simulink model "control_system"  (R2016b)
settings: Solver=FixedStepDiscrete  StartTime=0.0  StopTime=inf  FixedStep=0.004  MaxStep=0.004  RelTol=1e-3
undefined symbols (not defined in the file or in its folder): DiscIntNeverNeededParam
libraries: simulink x11
settings Model: Creator=ADAM  LastModifiedBy=consti
settings SolverCC: ExtrapolationOrder=1
settings DataIOCC: MaxDataPoints=1  SaveFormat=Structure  SignalLoggingSaveFormat=ModelDataLogs  SaveOutput=off  DSMLogging=off  SaveTime=off  OutputSaveName=model_out  SignalLoggingName=model_out
settings OptimizationCC: DefaultParameterBehavior=Inlined  UseFloatMulNetSlope=on  InlineInvariantSignals=on  PassReuseOutputArgsAs=Individual arguments  ExpressionDepthLimit=2147483647  ZeroExternalMemoryAtStartup=off  ZeroInternalMemoryAtStartup=off  NoFixptDivByZeroProtection=on  EfficientFloat2IntCast=on  LifeSpan=1
settings DebuggingCC: UnderspecifiedInitializationDetection=Classic  MergeDetectMultiDrivingBlocksExec=none  SolverPrmCheckMsg=warning  InheritedTsInSrcMsg=none  MultiTaskDSMMsg=warning  MultiTaskCondExecSysMsg=none  ParameterTunabilityLossMsg=error  UnconnectedInputMsg=none  UnconnectedOutputMsg=none  UnconnectedLineMsg=none  StateNameClashWarn=warning  SFUnexpectedBacktrackingDiag=warning  SFNoUnconditionalDefaultTransitionDiag=warning  SFExecutionAtInitializationDiag=none
settings HardwareCC: ProdBitPerLong=64  ProdHWDeviceType=Intel->x86-64 (Linux 64)
settings ModelReferenceCC: PropagateSignalLabelsOutOfModel=off
settings RTWCC: SystemTargetFile=ert.tlc  TemplateMakefile=ert_default_tmf  Description=Embedded Coder  GenerateReport=on  IncludeHyperlinkInReport=on  LaunchReport=on  GenerateTraceInfo=on  GenerateTraceReport=on  GenerateTraceReportSl=on  GenerateTraceReportSf=on  GenerateTraceReportEml=on  GenerateCodeMetricsReport=on
settings CodeAppCC: ForceParamTrailComments=on  IgnoreCustomStorageClasses=off  MaxIdLength=95  OperatorAnnotations=on  SimulinkDataObjDesc=on  SFDataObjDesc=on  MATLABFcnDesc=on  CustomSymbolStrGlobalVar=rt$N$M  CustomSymbolStrType=$N$M  CustomSymbolStrFcn=$N$M$F  CustomSymbolStrMacro=$N$M  InsertBlockDesc=on  MATLABSourceComments=on
settings ERTTargetCC: GenerateSampleERTMain=on  CombineSignalStateStructs=on  SupportAbsoluteTime=off  SupportComplex=off  SupportNonInlinedSFcns=on  InlinedParameterPlacement=NonHierarchical  ERTCustomFileTemplate=example_file_process.tlc  ERTFilePackagingFormat=CompactWithDataFile
settings ConfigComp: CovMetricSettings=dw  CovHtmlReporting=on  CovSaveCumulativeToWorkspaceVar=on  CovSaveSingleToWorkspaceVar=on  CovExternalEMLEnable=off  CovSFcnEnable=off

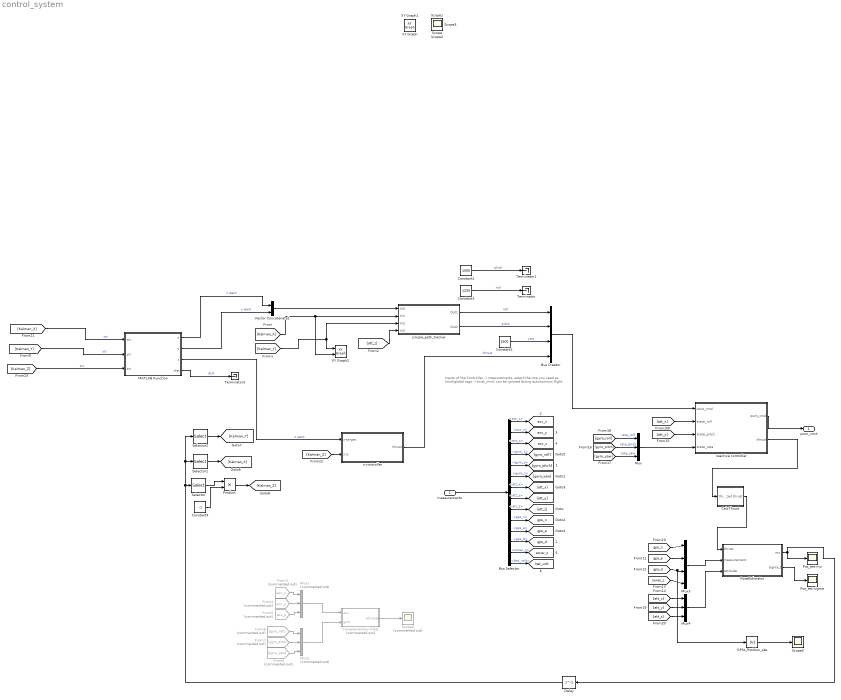
== system control_system ==
  note: Inputs of the Controller
      | -) measurements: select the one you need as local/global tags
      | -) twist_cmd: can be ignored during autonomous flight
  measurements : Inport  OutDataTypeStr=Bus: Sensor_Bus  SampleTime=[0.0040000000000000001,0]
  Bus Creator : BusCreator  Inputs=4
  Bus Selector : BusSelector  OutputSignals=acc_x,acc_y,acc_z,gyro_x,gyro_y,gyro_z,att_x,att_y,att_z,gps_n,gps_e,gps_d,sonar_z,bat_volt
  "CalcThrust " : MATLAB Function  TreatAsAtomicUnit=on
  Complementary Filter : Subsystem  Commented=on
  Constant1 : Constant  Value=1500
  Constant2 : Constant  Value=1500
  Constant3 : Constant  Value=1250
  Constant4 : Constant  Value=-1
  Delay : Delay  DelayLength=1  InitialCondition=0
  From3 : From  Commented=on  GotoTag=acc_x  TagVisibility=global
  From4 : From  Commented=on  GotoTag=acc_y  TagVisibility=global
  From5 : From  Commented=on  GotoTag=acc_z  TagVisibility=global
  From6 : From  Commented=on  GotoTag=gyro_roll
  From7 : From  Commented=on  GotoTag=gyro_pitch
  From8 : From  Commented=on  GotoTag=gyro_yaw
  GPSz_Position_abs : Abs
  MATLAB Function : MATLAB Function  TreatAsAtomicUnit=on
  Mux : Mux  Inputs=3
  Mux1 : Mux  Commented=on  Inputs=3
  Mux2 : Mux  Commented=on  Inputs=3
  Mux3 : Mux
  Mux4 : Mux  Inputs=3
  Pos_est-mu : Scope
  Pos_est-sigma : Scope
  "PoseEstimator " : MATLAB Function  TreatAsAtomicUnit=on
  Product : Product
  Scope4 : Scope  Commented=on
  Scope{,1..3,5} (5 alike) : Scope
  Selector : Selector  InputPortWidth=6  IndexOptions=Index vector (dialog)  Indices=[3]  OutputSizes=1
  Selector1 : Selector  InputPortWidth=6  IndexOptions=Index vector (dialog)  Indices=[2]  OutputSizes=1
  Selector2 : Selector  InputPortWidth=6  IndexOptions=Index vector (dialog)  Indices=[1]  OutputSizes=1
  Terminator : Terminator
  Terminator1 : Terminator
  Terminator3 : Terminator
  Vector Concatenate1 : Concatenate
  XY Graph2 : simulink/Sinks/XY Graph  xmin=0  xmax=20  ymin=0  ymax=20  st=-1
  reactive controller : Subsystem  TreatAsAtomicUnit=on
  "simple_path_tracker " : Subsystem
  z-controller : Subsystem
  pwm_cmd : Outport  OutDataTypeStr=Bus: Motor_Bus  SampleTime=[0.0040000000000000001,0]
  XY Graph : simulink/Sinks/XY Graph  IOType=viewer  xmin=-1  xmax=1  ymin=-1  ymax=1  st=-1
  XY Graph1 : simulink/Sinks/XY Graph  IOType=viewer  xmin=-1  xmax=1  ymin=-1  ymax=1  st=-1
  tag scope: acc_x=global, acc_y=global, acc_z=global, bat_volt=global, gps_d=global, gps_e=global, gps_n=global, sonar_z=global
  wires:
  reactive controller/1(pwm_cmd) -> pwm_cmd/1
  measurements/1 -> Bus Selector/1
  Mux/1 -> reactive controller/4(state_rate)
  [gyro_yaw] -> Mux/3  "rate_yaw"
  [gyro_pitch] -> Mux/2  "rate_pitch"
  [gyro_roll] -> Mux/1  "rate_roll"
  [att_y] -> reactive controller/3(state_pitch)
  [att_x] -> reactive controller/2(state_roll)
  Bus Selector/1 -> [acc_x]  "<acc_x>"
  Bus Selector/2 -> [acc_y]  "<acc_y>"
  Bus Selector/3 -> [acc_z]  "<acc_z>"
  Bus Selector/7 -> [att_x]  "<att_x>"
  Bus Selector/8 -> [att_y]  "<att_y>"
  Bus Selector/9 -> [att_z]  "<att_z>"
  Bus Selector/10 -> [gps_n]  "<gps_n>"
  Bus Selector/11 -> [gps_e]  "<gps_e>"
  Bus Selector/12 -> [gps_d]  "<gps_d>"
  Bus Selector/13 -> [sonar_z]  "<sonar_z>"
  Bus Selector/14 -> [bat_volt]  "<bat_volt>"
  Bus Selector/4 -> [gyro_roll]  "<gyro_x>"
  Bus Selector/5 -> [gyro_pitch]  "<gyro_y>"
  Bus Selector/6 -> [gyro_yaw]  "<gyro_z>"
  Bus Creator/1 -> reactive controller/1(twist_cmd)
  Constant1/1 -> Bus Creator/3  "yaw"
  z-controller/1(thrust) -> Bus Creator/4  "thrust"
  Vector Concatenate1/1 -> "simple_path_tracker "/1(In4)
  MATLAB Function/1(x) -> Vector Concatenate1/1  "x want"
  [Kalman_X] -> "simple_path_tracker "/2(In1), XY Graph2/2
  [Kalman_Y] -> "simple_path_tracker "/3(In2), XY Graph2/1
  MATLAB Function/2(y) -> Vector Concatenate1/2  "y want"
  [att_z] -> "simple_path_tracker "/4(In3)
  From3/1 -> Mux1/1
  From4/1 -> Mux1/2
  From5/1 -> Mux1/3
  Mux1/1 -> Complementary Filter/1(acc)
  From6/1 -> Mux2/1
  From7/1 -> Mux2/2
  From8/1 -> Mux2/3
  Mux2/1 -> Complementary Filter/2(gyro)
  Complementary Filter/1(attitude) -> Scope4/1
  MATLAB Function/3(z) -> z-controller/1(z-target)  "z want"
  [gps_n] -> Mux3/1
  [gps_e] -> Mux3/2
  [sonar_z] -> Mux3/4
  Mux3/1 -> "PoseEstimator "/2(measurement)
  [att_y] -> Mux4/2
  [att_x] -> Mux4/1
  [att_z] -> Mux4/3
  Mux4/1 -> "PoseEstimator "/3(attitude)
  "PoseEstimator "/2(sigma_t) -> Pos_est-sigma/1
  "CalcThrust "/1(thrust) -> "PoseEstimator "/1(thrust)
  reactive controller/2(thrust) -> "CalcThrust "/1(thrust_normalized)
  [gps_d] -> GPSz_Position_abs/1, Mux3/3
  GPSz_Position_abs/1 -> Scope5/1
  "PoseEstimator "/1(mu) -> Pos_est-mu/1, Delay/1
  Delay/1 -> Selector2/1, Selector1/1, Selector/1
  Selector/1 -> Product/1
  Constant4/1 -> Product/2
  Constant2/1 -> Terminator1/1  "pitch"
  Constant3/1 -> Terminator/1  "roll"
  [Kalman_Y] -> MATLAB Function/2(yis)  "yis"
  [Kalman_X] -> MATLAB Function/1(xis)  "xis"
  [Kalman_Z] -> MATLAB Function/3(zis)  "zis"
  "simple_path_tracker "/1(Out1) -> Bus Creator/1  "roll"
  "simple_path_tracker "/2(Out2) -> Bus Creator/2  "pitch"
  MATLAB Function/4(dist) -> Terminator3/1  "dist"
  Selector1/1 -> [Kalman_X]
  Selector2/1 -> [Kalman_Y]
  Product/1 -> [Kalman_Z]
  [Kalman_Z] -> z-controller/2(z-is)

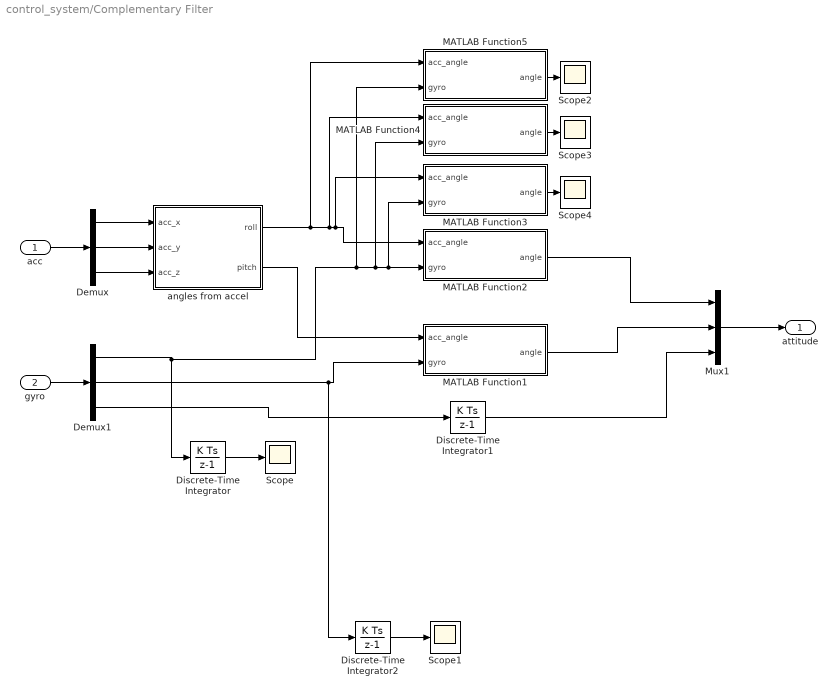
== system control_system/Complementary Filter ==
  acc : Inport  PortDimensions=3
  gyro : Inport  Port=2
  Demux : Demux  Outputs=3
  Demux1 : Demux  Outputs=3
  Discrete-Time Integrator : DiscreteIntegrator  InitialConditionSetting=State (most efficient)  SampleTime=-1  ICPrevOutput=DiscIntNeverNeededParam  ICPrevScaledInput=DiscIntNeverNeededParam
  Discrete-Time Integrator1 : DiscreteIntegrator  InitialConditionSetting=State (most efficient)  SampleTime=-1  ICPrevOutput=DiscIntNeverNeededParam  ICPrevScaledInput=DiscIntNeverNeededParam
  Discrete-Time Integrator2 : DiscreteIntegrator  InitialConditionSetting=State (most efficient)  SampleTime=-1  ICPrevOutput=DiscIntNeverNeededParam  ICPrevScaledInput=DiscIntNeverNeededParam
  MATLAB Function1 : MATLAB Function  TreatAsAtomicUnit=on
  MATLAB Function2 : MATLAB Function  TreatAsAtomicUnit=on
  MATLAB Function3 : MATLAB Function  TreatAsAtomicUnit=on
  MATLAB Function4 : MATLAB Function  TreatAsAtomicUnit=on
  MATLAB Function5 : MATLAB Function  TreatAsAtomicUnit=on
  Mux1 : Mux  Inputs=3
  Scope{,1..4} (5 alike) : Scope
  angles from accel : MATLAB Function  TreatAsAtomicUnit=on
  attitude : Outport
  wires:
  Mux1/1 -> attitude/1
  acc/1 -> Demux/1
  gyro/1 -> Demux1/1
  Demux/1 -> angles from accel/1(acc_x)
  Demux/3 -> angles from accel/3(acc_z)
  Demux/2 -> angles from accel/2(acc_y)
  angles from accel/2(pitch) -> MATLAB Function1/1(acc_angle)
  MATLAB Function1/1(angle) -> Mux1/2
  Discrete-Time Integrator/1 -> Scope/1
  angles from accel/1(roll) -> MATLAB Function5/1(acc_angle), MATLAB Function4/1(acc_angle), MATLAB Function3/1(acc_angle), MATLAB Function2/1(acc_angle)
  MATLAB Function2/1(angle) -> Mux1/1
  Demux1/3 -> Discrete-Time Integrator1/1
  Discrete-Time Integrator1/1 -> Mux1/3
  Demux1/2 -> Discrete-Time Integrator2/1, MATLAB Function1/2(gyro)
  Discrete-Time Integrator2/1 -> Scope1/1
  Demux1/1 -> MATLAB Function5/2(gyro), MATLAB Function4/2(gyro), MATLAB Function2/2(gyro), MATLAB Function3/2(gyro), Discrete-Time Integrator/1
  MATLAB Function5/1(angle) -> Scope2/1
  MATLAB Function4/1(angle) -> Scope3/1
  MATLAB Function3/1(angle) -> Scope4/1

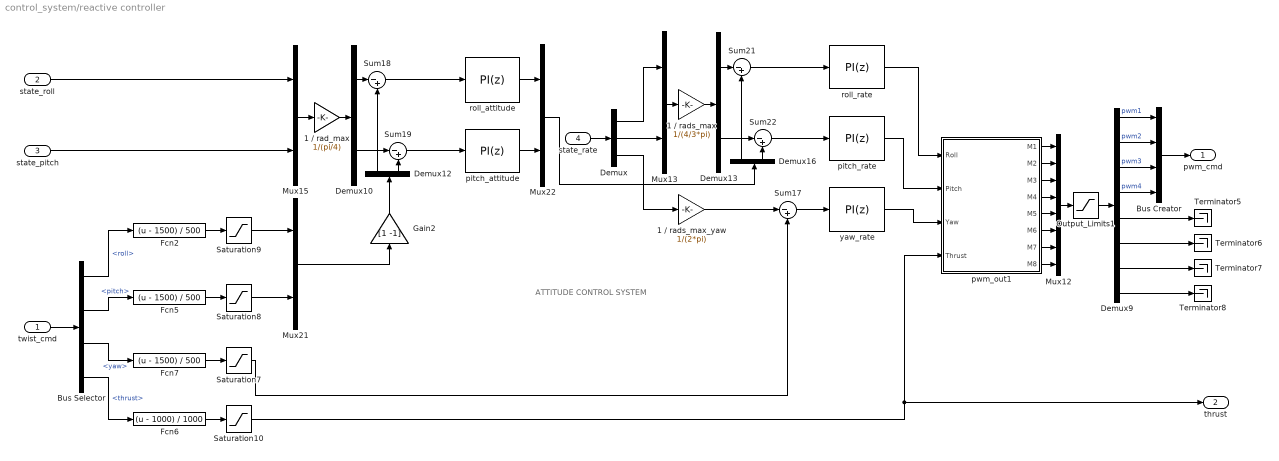
== system control_system/reactive controller ==
  note: ATTITUDE CONTROL SYSTEM
  twist_cmd : Inport  OutDataTypeStr=Bus: Twist_Bus
  state_roll : Inport  Port=2
  state_pitch : Inport  Port=3
  state_rate : Inport  Port=4
  1 / rad_max : Gain  Gain=1/(pi/4)
  1 / rads_max : Gain  Gain=1/(4/3*pi)
  1 / rads_max_yaw : Gain  Gain=1/(2*pi)
  Bus Creator : BusCreator  Inputs=4
  Bus Selector : BusSelector  OutputSignals=roll,pitch,yaw,thrust
  Demux : Demux  Outputs=3
  Demux{10,12..13,16} (4 alike) : Demux  Outputs=2
  Demux9 : Demux  Outputs=8
  Fcn2 : Fcn  Expr=(u - 1500) / 500
  Fcn5 : Fcn  Expr=(u - 1500) / 500
  Fcn6 : Fcn  Expr=(u - 1000) / 1000
  Fcn7 : Fcn  Expr=(u - 1500) / 500
  Gain2 : Gain  Gain=[1 -1]
  Mux12 : Mux  Inputs=8
  Mux{13,15,21..22} (4 alike) : Mux  Inputs=2
  Output_Limits1 : Saturate  UpperLimit=2000  LowerLimit=1000
  Saturation10 : Saturate  UpperLimit=1  LowerLimit=0
  Saturation7 : Saturate  UpperLimit=1  LowerLimit=-1
  Saturation8 : Saturate  UpperLimit=1  LowerLimit=-1
  Saturation9 : Saturate  UpperLimit=1  LowerLimit=-1
  Sum{17..19,21..22} (5 alike) : Sum  Inputs=|-+
  Terminator{5..8} (4 alike) : Terminator
  pitch_attitude : simulink/Continuous/PID Controller  Controller=PI  TimeDomain=Discrete-time  SampleTime=-1  IntegratorMethod=Forward Euler  FilterMethod=Forward Euler  Form=Parallel  UseFilter=on  ControllerParametersSource=internal  P=0.5  I=0.05  D=0.01  N=100  InitialConditionSource=internal  InitialConditionForIntegrator=0  InitialConditionForFilter=0  ExternalReset=none  LimitOutput=on  UpperSaturationLimit=1  LowerSaturationLimit=-1  LinearizeAsGain=on  AntiWindupMode=none  Kb=1  TrackingMode=off  Kt=1  PParamMin=[]  PParamMax=[]  IParamMin=[]  IParamMax=[]  DParamMin=[]  DParamMax=[]  NParamMin=[]  NParamMax=[]  KbParamMin=[]  KbParamMax=[]  KtParamMin=[]  KtParamMax=[]  POutMin=[]  POutMax=[]  IOutMin=[]  IOutMax=[]  DOutMin=[]  DOutMax=[]  NOutMin=[]  NOutMax=[]  KbOutMin=[]  KbOutMax=[]  KtOutMin=[]  KtOutMax=[]  IntegratorOutMin=[]  IntegratorOutMax=[]  FilterOutMin=[]  FilterOutMax=[]  SumOutMin=[]  SumOutMax=[]  SumI1OutMin=[]  SumI1OutMax=[]  SumI2OutMin=[]  SumI2OutMax=[]  SumI3OutMin=[]  SumI3OutMax=[]  SumDOutMin=[]  SumDOutMax=[]  SaturationOutMin=[]  SaturationOutMax=[]  IntegratorContinuousStateAttributes=''  IntegratorStateMustResolveToSignalObject=off  IntegratorRTWStateStorageClass=Auto  FilterContinuousStateAttributes=''  FilterStateMustResolveToSignalObject=off  FilterRTWStateStorageClass=Auto  DifferentiatorICPrevScaledInput=0  DifferentiatorOutMin=[]  DifferentiatorOutMax=[]
  pitch_rate : simulink/Continuous/PID Controller  Controller=PI  TimeDomain=Discrete-time  SampleTime=-1  IntegratorMethod=Forward Euler  FilterMethod=Forward Euler  Form=Parallel  UseFilter=on  ControllerParametersSource=internal  P=0.3  I=0.03  D=0.0024  N=100  InitialConditionSource=internal  InitialConditionForIntegrator=0  InitialConditionForFilter=0  ExternalReset=none  LimitOutput=on  UpperSaturationLimit=1  LowerSaturationLimit=-1  LinearizeAsGain=on  AntiWindupMode=none  Kb=1  TrackingMode=off  Kt=1  PParamMin=[]  PParamMax=[]  IParamMin=[]  IParamMax=[]  DParamMin=[]  DParamMax=[]  NParamMin=[]  NParamMax=[]  KbParamMin=[]  KbParamMax=[]  KtParamMin=[]  KtParamMax=[]  POutMin=[]  POutMax=[]  IOutMin=[]  IOutMax=[]  DOutMin=[]  DOutMax=[]  NOutMin=[]  NOutMax=[]  KbOutMin=[]  KbOutMax=[]  KtOutMin=[]  KtOutMax=[]  IntegratorOutMin=[]  IntegratorOutMax=[]  FilterOutMin=[]  FilterOutMax=[]  SumOutMin=[]  SumOutMax=[]  SumI1OutMin=[]  SumI1OutMax=[]  SumI2OutMin=[]  SumI2OutMax=[]  SumI3OutMin=[]  SumI3OutMax=[]  SumDOutMin=[]  SumDOutMax=[]  SaturationOutMin=[]  SaturationOutMax=[]  IntegratorContinuousStateAttributes=''  IntegratorStateMustResolveToSignalObject=off  IntegratorRTWStateStorageClass=Auto  FilterContinuousStateAttributes=''  FilterStateMustResolveToSignalObject=off  FilterRTWStateStorageClass=Auto  DifferentiatorICPrevScaledInput=0  DifferentiatorOutMin=[]  DifferentiatorOutMax=[]
  pwm_out1 : MATLAB Function  TreatAsAtomicUnit=on  SystemSampleTime=0.004
  roll_attitude : simulink/Continuous/PID Controller  Controller=PI  TimeDomain=Discrete-time  SampleTime=-1  IntegratorMethod=Forward Euler  FilterMethod=Forward Euler  Form=Parallel  UseFilter=on  ControllerParametersSource=internal  P=0.5  I=0.05  D=0.01  N=100  InitialConditionSource=internal  InitialConditionForIntegrator=0  InitialConditionForFilter=0  ExternalReset=none  LimitOutput=on  UpperSaturationLimit=1  LowerSaturationLimit=-1  LinearizeAsGain=on  AntiWindupMode=none  Kb=1  TrackingMode=off  Kt=1  PParamMin=[]  PParamMax=[]  IParamMin=[]  IParamMax=[]  DParamMin=[]  DParamMax=[]  NParamMin=[]  NParamMax=[]  KbParamMin=[]  KbParamMax=[]  KtParamMin=[]  KtParamMax=[]  POutMin=[]  POutMax=[]  IOutMin=[]  IOutMax=[]  DOutMin=[]  DOutMax=[]  NOutMin=[]  NOutMax=[]  KbOutMin=[]  KbOutMax=[]  KtOutMin=[]  KtOutMax=[]  IntegratorOutMin=[]  IntegratorOutMax=[]  FilterOutMin=[]  FilterOutMax=[]  SumOutMin=[]  SumOutMax=[]  SumI1OutMin=[]  SumI1OutMax=[]  SumI2OutMin=[]  SumI2OutMax=[]  SumI3OutMin=[]  SumI3OutMax=[]  SumDOutMin=[]  SumDOutMax=[]  SaturationOutMin=[]  SaturationOutMax=[]  IntegratorContinuousStateAttributes=''  IntegratorStateMustResolveToSignalObject=off  IntegratorRTWStateStorageClass=Auto  FilterContinuousStateAttributes=''  FilterStateMustResolveToSignalObject=off  FilterRTWStateStorageClass=Auto  DifferentiatorICPrevScaledInput=0  DifferentiatorOutMin=[]  DifferentiatorOutMax=[]
  roll_rate : simulink/Continuous/PID Controller  Controller=PI  TimeDomain=Discrete-time  SampleTime=-1  IntegratorMethod=Forward Euler  FilterMethod=Forward Euler  Form=Parallel  UseFilter=on  ControllerParametersSource=internal  P=0.3  I=0.03  D=0.0024  N=100  InitialConditionSource=internal  InitialConditionForIntegrator=0  InitialConditionForFilter=0  ExternalReset=none  LimitOutput=on  UpperSaturationLimit=1  LowerSaturationLimit=-1  LinearizeAsGain=on  AntiWindupMode=none  Kb=1  TrackingMode=off  Kt=1  PParamMin=[]  PParamMax=[]  IParamMin=[]  IParamMax=[]  DParamMin=[]  DParamMax=[]  NParamMin=[]  NParamMax=[]  KbParamMin=[]  KbParamMax=[]  KtParamMin=[]  KtParamMax=[]  POutMin=[]  POutMax=[]  IOutMin=[]  IOutMax=[]  DOutMin=[]  DOutMax=[]  NOutMin=[]  NOutMax=[]  KbOutMin=[]  KbOutMax=[]  KtOutMin=[]  KtOutMax=[]  IntegratorOutMin=[]  IntegratorOutMax=[]  FilterOutMin=[]  FilterOutMax=[]  SumOutMin=[]  SumOutMax=[]  SumI1OutMin=[]  SumI1OutMax=[]  SumI2OutMin=[]  SumI2OutMax=[]  SumI3OutMin=[]  SumI3OutMax=[]  SumDOutMin=[]  SumDOutMax=[]  SaturationOutMin=[]  SaturationOutMax=[]  IntegratorContinuousStateAttributes=''  IntegratorStateMustResolveToSignalObject=off  IntegratorRTWStateStorageClass=Auto  FilterContinuousStateAttributes=''  FilterStateMustResolveToSignalObject=off  FilterRTWStateStorageClass=Auto  DifferentiatorICPrevScaledInput=0  DifferentiatorOutMin=[]  DifferentiatorOutMax=[]
  yaw_rate : simulink/Continuous/PID Controller  Controller=PI  TimeDomain=Discrete-time  SampleTime=-1  IntegratorMethod=Forward Euler  FilterMethod=Forward Euler  Form=Parallel  UseFilter=on  ControllerParametersSource=internal  P=0.5  I=0.05  D=0  N=100  InitialConditionSource=internal  InitialConditionForIntegrator=0  InitialConditionForFilter=0  ExternalReset=none  LimitOutput=on  UpperSaturationLimit=1  LowerSaturationLimit=-1  LinearizeAsGain=on  AntiWindupMode=none  Kb=1  TrackingMode=off  Kt=1  PParamMin=[]  PParamMax=[]  IParamMin=[]  IParamMax=[]  DParamMin=[]  DParamMax=[]  NParamMin=[]  NParamMax=[]  KbParamMin=[]  KbParamMax=[]  KtParamMin=[]  KtParamMax=[]  POutMin=[]  POutMax=[]  IOutMin=[]  IOutMax=[]  DOutMin=[]  DOutMax=[]  NOutMin=[]  NOutMax=[]  KbOutMin=[]  KbOutMax=[]  KtOutMin=[]  KtOutMax=[]  IntegratorOutMin=[]  IntegratorOutMax=[]  FilterOutMin=[]  FilterOutMax=[]  SumOutMin=[]  SumOutMax=[]  SumI1OutMin=[]  SumI1OutMax=[]  SumI2OutMin=[]  SumI2OutMax=[]  SumI3OutMin=[]  SumI3OutMax=[]  SumDOutMin=[]  SumDOutMax=[]  SaturationOutMin=[]  SaturationOutMax=[]  IntegratorContinuousStateAttributes=''  IntegratorStateMustResolveToSignalObject=off  IntegratorRTWStateStorageClass=Auto  FilterContinuousStateAttributes=''  FilterStateMustResolveToSignalObject=off  FilterRTWStateStorageClass=Auto  DifferentiatorICPrevScaledInput=0  DifferentiatorOutMin=[]  DifferentiatorOutMax=[]
  pwm_cmd : Outport  OutDataTypeStr=Bus: Motor_Bus
  thrust : Outport  Port=2
  wires:
  Demux/3 -> 1 / rads_max_yaw/1
  Demux/1 -> Mux13/1
  Bus Creator/1 -> pwm_cmd/1
  state_pitch/1 -> Mux15/2
  state_roll/1 -> Mux15/1
  Bus Selector/4 -> Fcn6/1  "<thrust>"
  Bus Selector/3 -> Fcn7/1  "<yaw>"
  Bus Selector/2 -> Fcn5/1  "<pitch>"
  twist_cmd/1 -> Bus Selector/1
  pwm_out1/2(M2) -> Mux12/2
  Fcn2/1 -> Saturation9/1
  Demux9/5 -> Terminator5/1
  yaw_rate/1 -> pwm_out1/3(Yaw)
  Demux16/2 -> Sum22/2
  pwm_out1/4(M4) -> Mux12/4
  Mux21/1 -> Gain2/1
  Sum21/1 -> roll_rate/1
  pwm_out1/5(M5) -> Mux12/5
  pitch_rate/1 -> pwm_out1/2(Pitch)
  Demux12/1 -> Sum18/2
  pwm_out1/8(M8) -> Mux12/8
  Saturation8/1 -> Mux21/2
  1 / rads_max_yaw/1 -> Sum17/1
  Fcn6/1 -> Saturation10/1
  1 / rads_max/1 -> Demux13/1
  Demux13/2 -> Sum22/1
  Sum17/1 -> yaw_rate/1
  Saturation7/1 -> Sum17/2
  Demux9/2 -> Bus Creator/2  "pwm2"
  Demux9/7 -> Terminator7/1
  Demux9/4 -> Bus Creator/4  "pwm4"
  pitch_attitude/1 -> Mux22/2
  Mux13/1 -> 1 / rads_max/1
  Mux12/1 -> Output_Limits1/1
  Mux15/1 -> 1 / rad_max/1
  Saturation10/1 -> thrust/1, pwm_out1/4(Thrust)
  roll_attitude/1 -> Mux22/1
  pwm_out1/6(M6) -> Mux12/6
  Demux9/1 -> Bus Creator/1  "pwm1"
  Fcn7/1 -> Saturation7/1
  pwm_out1/3(M3) -> Mux12/3
  Demux13/1 -> Sum21/1
  Sum22/1 -> pitch_rate/1
  Fcn5/1 -> Saturation8/1
  Gain2/1 -> Demux12/1
  Sum19/1 -> pitch_attitude/1
  Demux9/6 -> Terminator6/1
  1 / rad_max/1 -> Demux10/1
  Demux12/2 -> Sum19/2
  Mux22/1 -> Demux16/1
  Saturation9/1 -> Mux21/1
  pwm_out1/7(M7) -> Mux12/7
  pwm_out1/1(M1) -> Mux12/1
  Sum18/1 -> roll_attitude/1
  Output_Limits1/1 -> Demux9/1
  Demux9/3 -> Bus Creator/3  "pwm3"
  Demux16/1 -> Sum21/2
  roll_rate/1 -> pwm_out1/1(Roll)
  Demux10/1 -> Sum18/1
  Demux9/8 -> Terminator8/1
  Demux10/2 -> Sum19/1
  Demux/2 -> Mux13/2
  state_rate/1 -> Demux/1
  Bus Selector/1 -> Fcn2/1  "<roll>"

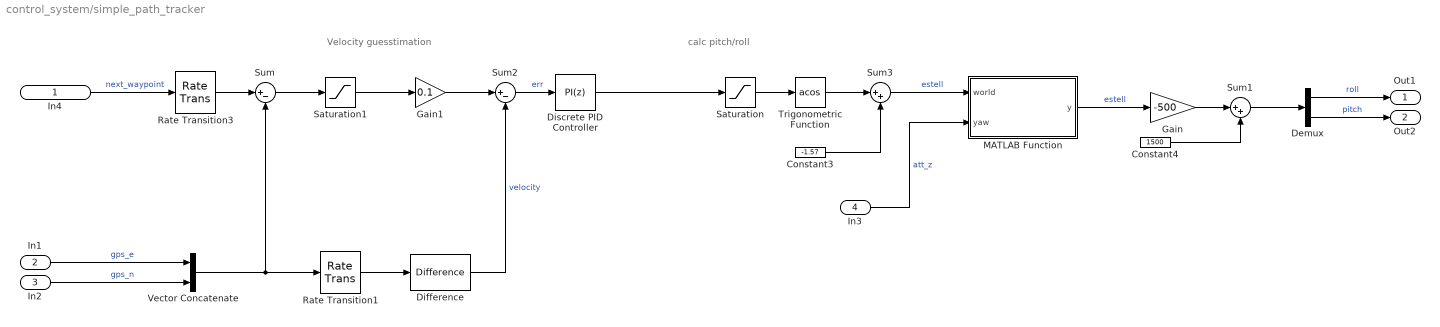
== system control_system/simple_path_tracker  ==
  note: calc pitch/roll
  note: Velocity guesstimation
  In4 : Inport
  In1 : Inport  Port=2
  In2 : Inport  Port=3
  In3 : Inport  Port=4
  Constant3 : Constant  Value=-1.57
  Constant4 : Constant  Value=1500
  Demux : Demux  Outputs=2
  Difference : simulink/Discrete/Difference  ICPrevInput=0.0  OutMin=[]  OutMax=[]  OutDataType=fixdt(1, 16)  OutScaling=2^-10  DoSatur=off
  Discrete PID Controller : simulink/Continuous/PID Controller  Controller=PI  TimeDomain=Discrete-time  SampleTime=-1  IntegratorMethod=Forward Euler  FilterMethod=Forward Euler  Form=Parallel  UseFilter=on  ControllerParametersSource=internal  P=1.2*0.45  I=1.2*0.45/3.1  D=0  N=1000  InitialConditionSource=internal  InitialConditionForIntegrator=0  InitialConditionForFilter=0  ExternalReset=none  LimitOutput=off  UpperSaturationLimit=inf  LowerSaturationLimit=-inf  LinearizeAsGain=off  AntiWindupMode=none  Kb=1  TrackingMode=off  Kt=1  PParamMin=[]  PParamMax=[]  IParamMin=[]  IParamMax=[]  DParamMin=[]  DParamMax=[]  NParamMin=[]  NParamMax=[]  KbParamMin=[]  KbParamMax=[]  KtParamMin=[]  KtParamMax=[]  POutMin=[]  POutMax=[]  IOutMin=[]  IOutMax=[]  DOutMin=[]  DOutMax=[]  NOutMin=[]  NOutMax=[]  KbOutMin=[]  KbOutMax=[]  KtOutMin=[]  KtOutMax=[]  IntegratorOutMin=[]  IntegratorOutMax=[]  FilterOutMin=[]  FilterOutMax=[]  SumOutMin=[]  SumOutMax=[]  SumI1OutMin=[]  SumI1OutMax=[]  SumI2OutMin=[]  SumI2OutMax=[]  SumI3OutMin=[]  SumI3OutMax=[]  SumDOutMin=[]  SumDOutMax=[]  SaturationOutMin=[]  SaturationOutMax=[]  IntegratorContinuousStateAttributes=''  IntegratorStateMustResolveToSignalObject=off  IntegratorRTWStateStorageClass=Auto  FilterContinuousStateAttributes=''  FilterStateMustResolveToSignalObject=off  FilterRTWStateStorageClass=Auto  DifferentiatorICPrevScaledInput=0  DifferentiatorOutMin=[]  DifferentiatorOutMax=[]
  Gain : Gain  Gain=-500
  Gain1 : Gain  Gain=0.1
  MATLAB Function : MATLAB Function  TreatAsAtomicUnit=on
  Rate Transition1 : RateTransition  OutPortSampleTime=0.2
  Rate Transition3 : RateTransition  OutPortSampleTime=0.2
  Saturation : Saturate  UpperLimit=1  LowerLimit=-1
  Saturation1 : Saturate  UpperLimit=10  LowerLimit=-10
  Sum : Sum  Inputs=|+-
  Sum1 : Sum  Inputs=|++
  Sum2 : Sum  Inputs=|+-
  Sum3 : Sum  Inputs=|++
  Trigonometric Function : Trigonometry  Operator=acos
  Vector Concatenate : Concatenate
  Out1 : Outport
  Out2 : Outport  Port=2
  wires:
  Constant4/1 -> Sum1/2
  Gain/1 -> Sum1/1
  Saturation/1 -> Trigonometric Function/1
  Sum/1 -> Saturation1/1
  Saturation1/1 -> Gain1/1
  Sum2/1 -> Discrete PID Controller/1  "err"
  Rate Transition1/1 -> Difference/1
  Constant3/1 -> Sum3/2
  MATLAB Function/1(y) -> Gain/1  "estell"
  Gain1/1 -> Sum2/1
  Difference/1 -> Sum2/2  "velocity"
  In1/1 -> Vector Concatenate/1  "gps_e"
  In2/1 -> Vector Concatenate/2  "gps_n"
  Vector Concatenate/1 -> Rate Transition1/1, Sum/2
  Rate Transition3/1 -> Sum/1
  Discrete PID Controller/1 -> Saturation/1
  In3/1 -> MATLAB Function/2(yaw)  "att_z"
  Trigonometric Function/1 -> Sum3/1
  Sum3/1 -> MATLAB Function/1(world)  "estell"
  Demux/1 -> Out1/1  "roll"
  Demux/2 -> Out2/1  "pitch"
  Sum1/1 -> Demux/1
  In4/1 -> Rate Transition3/1  "next_waypoint"

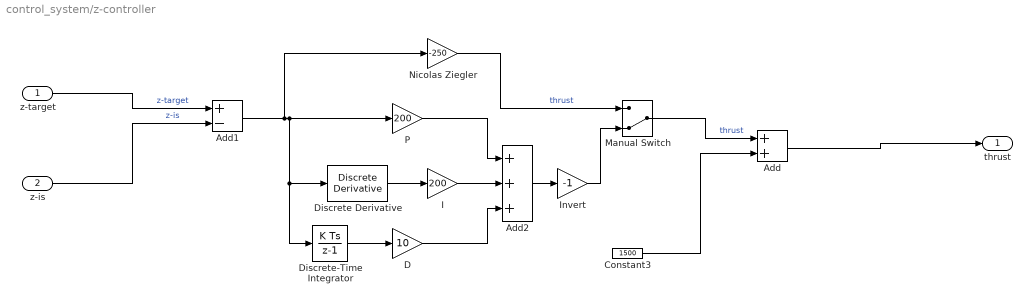
== system control_system/z-controller ==
  z-target : Inport
  z-is : Inport  Port=2
  Add : Sum
  Add1 : Sum  Inputs=+-
  Add2 : Sum  Inputs=+++
  Constant3 : Constant  Value=1500
  D : Gain  Gain=10
  Discrete Derivative : simulink/Discrete/Discrete Derivative  gainval=1.0  ICPrevScaledInput=0.0  OutMin=[]  OutMax=[]  OutDataType=fixdt(1, 16)  OutScaling=2^-10  DoSatur=off
  Discrete-Time Integrator : DiscreteIntegrator  InitialConditionSetting=State (most efficient)  ICPrevOutput=DiscIntNeverNeededParam  ICPrevScaledInput=DiscIntNeverNeededParam
  I : Gain  Gain=200
  Invert : Gain  Gain=-1
  Manual Switch : ManualSwitch  CurrentSetting=0
  Nicolas Ziegler : Gain  Gain=-250
  P : Gain  Gain=200
  thrust : Outport
  wires:
  Add1/1 -> P/1, Discrete-Time Integrator/1, Discrete Derivative/1, Nicolas Ziegler/1
  Discrete Derivative/1 -> I/1
  Discrete-Time Integrator/1 -> D/1
  D/1 -> Add2/3
  I/1 -> Add2/2
  Nicolas Ziegler/1 -> Manual Switch/1  "thrust"
  P/1 -> Add2/1
  Invert/1 -> Manual Switch/2
  Add2/1 -> Invert/1
  z-target/1 -> Add1/1  "z-target"
  z-is/1 -> Add1/2  "z-is"
  Manual Switch/1 -> Add/1  "thrust"
  Constant3/1 -> Add/2
  Add/1 -> thrust/1

== matlab function control_system/simple_path_tracker /MATLAB Function ==
  data: world input; y output; yaw input
function y = yawCorrection(world,yaw)

y = zeros(2,1);
y(1)=world(1)*cos(yaw)-world(2)*sin(yaw);
y(2)=world(1)*sin(yaw)+world(2)*cos(yaw);

== matlab function control_system/Complementary Filter/MATLAB Function2 ==
  data: acc_angle input; angle output; gyro input
function angle = complementary_filter(acc_angle, gyro)
alpha = 0.99999;
dt = 0.004;

persistent prev_angle;
if isempty(prev_angle)
    prev_angle = 0;
end

new_angle = alpha * (prev_angle + gyro * dt) + (1-alpha) * acc_angle;
prev_angle = new_angle;
angle = new_angle;

== matlab function control_system/Complementary Filter/angles from accel ==
  data: acc_x input; roll output; acc_y input; acc_z input; pitch output
function [roll, pitch] = angles_from_accel(acc_x, acc_y, acc_z)
roll_n = atan2(acc_y, sqrt(acc_z^2+acc_x^2));
if (roll_n > pi)
    roll_n = roll_n - 2*pi;
end
roll = -roll_n;
pitch_n = atan2(acc_x, sqrt(acc_z^2+acc_y^2));
if (pitch_n > pi)
    pitch_n = pitch_n - 2*pi;
end
pitch = pitch_n;

== matlab function control_system/reactive controller/pwm_out1 ==
  data: Roll input; M1 output; Pitch input; Yaw input; Thrust input; M2 output; M3 output; M4 output; M5 output; M6 output; M7 output; M8 output
function [M1, M2, M3, M4, M5, M6, M7, M8] = motor_mixer(Roll, Pitch, Yaw, Thrust)

idle_PWM = 1000;

% Quad X
M1 = ((Roll + Pitch - Yaw) / 2 * Thrust + Thrust) * 1000 + idle_PWM;
M2 = ((-Roll + Pitch + Yaw) / 2 * Thrust + Thrust) * 1000 + idle_PWM;
M3 = ((-Roll - Pitch - Yaw) / 2 * Thrust + Thrust) * 1000 + idle_PWM;
M4 = ((Roll - Pitch + Yaw) / 2 * Thrust + Thrust) * 1000 + idle_PWM;
M5 = 1000;
M6 = 1000;
M7 = 1000;
M8 = 1000;

% Quad +
% M1 = ((Pitch - Yaw) * Thrust / 2 + Thrust) * 1000 + idle_PWM;
% M2 = ((-Roll + Yaw) * Thrust / 2 + Thrust) * 1000 + idle_PWM;
% M3 = ((-Pitch - Yaw) * Thrust / 2 + Thrust) * 1000 + idle_PWM;
% M4 = ((Roll + Yaw) * Thrust / 2 + Thrust) * 1000 + idle_PWM;
% M5 = 1000;
% M6 = 1000;
% M7 = 1000;
% M8 = 1000;

% Hex X
% M1 = ((Pitch + Roll / 2 - Yaw) * Thrust / 2 + Thrust) * 1000 + idle_PWM;
% M2 = ((Pitch - Roll / 2 + Yaw) * Thrust / 2 + Thrust) * 1000 + idle_PWM;
% M3 = ((-Roll - Yaw) * Thrust / 2 + Thrust) * 1000 + idle_PWM;
% M4 = ((-Pitch - Roll / 2 + Yaw) * Thrust / 2 + Thrust) * 1000 + idle_PWM;
% M5 = ((-Pitch + Roll / 2 - Yaw) * Thrust / 2 + Thrust) * 1000 + idle_PWM;
% M6 = ((Roll + Yaw) * Thrust / 2 + Thrust) * 1000 + idle_PWM;
% M7 = 1000;
% M8 = 1000;

== matlab function control_system/Complementary Filter/MATLAB Function1 ==
  data: acc_angle input; angle output; gyro input
function angle = complementary_filter(acc_angle, gyro)
alpha = 1;
dt = 0.004;

persistent prev_angle;
if isempty(prev_angle)
    prev_angle = 0;
end

new_angle = alpha * (prev_angle + gyro * dt) + (1-alpha) * acc_angle;
prev_angle = new_angle;
angle = new_angle;

== matlab function control_system/Complementary Filter/MATLAB Function3 ==
  data: acc_angle input; angle output; gyro input
function angle = complementary_filter(acc_angle, gyro)
alpha = 0.9999;
dt = 0.004;

persistent prev_angle;
if isempty(prev_angle)
    prev_angle = 0;
end

new_angle = alpha * (prev_angle + gyro * dt) + (1-alpha) * acc_angle;
prev_angle = new_angle;
angle = new_angle;

== matlab function control_system/Complementary Filter/MATLAB Function4 ==
  data: acc_angle input; angle output; gyro input
function angle = complementary_filter(acc_angle, gyro)
alpha = 0.999;
dt = 0.004;

persistent prev_angle;
if isempty(prev_angle)
    prev_angle = 0;
end

new_angle = alpha * (prev_angle + gyro * dt) + (1-alpha) * acc_angle;
prev_angle = new_angle;
angle = new_angle;

== matlab function control_system/Complementary Filter/MATLAB Function5 ==
  data: acc_angle input; angle output; gyro input
function angle = complementary_filter(acc_angle, gyro)
alpha = 0.99;
dt = 0.004;

persistent prev_angle;
if isempty(prev_angle)
    prev_angle = 0;
end

new_angle = alpha * (prev_angle + gyro * dt) + (1-alpha) * acc_angle;
prev_angle = new_angle;
angle = new_angle;

== matlab function control_system/CalcThrust  ==
  data: thrust_normalized input; thrust output
function thrust = CalcThrust(thrust_normalized)
%#codegen


maxAirVelocity = 70;               %TODO FIND MAX V through 1 rotor
air_density = 1.225;                     %kg/m^3
rotor_diameter = 0.1397;            % diameter of the propellor              (meters)   
%rotor_inertia = 0.0000025;          % rotor inertia (torque for angular acc) (kg m^2)                                  
%aircraft_diameter = 0.25;           % motor to motor distance               (meters)                                 
%aircraft_mass = 0.26;               % aircraft mass                         (kg)  

%thrust kg m /s^2


air_velocity = maxAirVelocity * thrust_normalized;
thrust = (pi/4 * rotor_diameter^2 * 4) * air_density * air_velocity;

== matlab function control_system/PoseEstimator  ==
  data: thrust input; mu output size=6; measurement input; sigma_t output; attitude input
function [mu, sigma_t] = pos_est(thrust, measurement, attitude)

%need to get t (simulation timestep)
t = 0.004;
t_sonar = 0.1;
t_gps = 0.2;
m = 0.26;
g = 9.81;

persistent x;
persistent sigma;
persistent t_act_sonar;
persistent t_act_gps;


if isempty(t_act_gps)
    t_act_gps = t_gps;
end
if isempty(t_act_sonar)
    t_act_sonar = t_sonar;
end

t_act_sonar = t_act_sonar + t;
t_act_gps = t_act_gps + t;


%DETECT MEASUREMENT CHANGED
persistent last_measurement;
if isempty(last_measurement)
    last_measurement = measurement;
end
if last_measurement(4) ~= measurement(4)
    t_act_sonar = t_act_sonar + t_sonar;
end
if (last_measurement(1) ~= measurement(1)) || (last_measurement(2) ~= measurement(2)) || (last_measurement(3) ~= measurement(3)) 
    t_act_gps = t_act_gps + t_gps;
end




if isempty(x)
    x = [0;
         0;
         1; %TODO: set start position
         0;
         0;
         0];
end
if isempty(sigma)
    sigma = [1e-8 0    0    0    0    0;
             0   1e-8  0    0    0    0;
             0    0   1e-8  0    0    0;
             0    0    0   1e-8  0    0;
             0    0    0    0   1e-8  0;
             0    0    0    0    0   1e-8];
end;


phi = -attitude(1);
theta = -attitude(2);
psi = attitude(3);

Kp = 0.282;       %todo tEST 

%TODO: some signs may be wrong here (different papers show them
%differently) - check in simulation
f_x = [x(4); 
       x(5); 
       x(6); 
       (cos(phi)*sin(theta)*cos(psi) + sin(phi)*sin(psi)) * (thrust - Kp * x(4))/m; 
       (cos(phi)*sin(theta)*sin(psi) - sin(phi)*cos(psi)) * (thrust - Kp * x(5))/m; 
       -g + cos(phi)*cos(theta)*(thrust - Kp * x(6))/m]; %note: z pointing upwards

G = [ 1 0 0 t 0 0;
      0 1 0 0 t 0;
      0 0 1 0 0 t;
      0 0 0 1 0 0;
      0 0 0 0 1 0;
      0 0 0 0 0 1];

%u is [phi theta psi thrust]'
v_4_1 = (sin(psi)*cos(phi)-sin(theta)*cos(psi)*sin(phi))*thrust/m;
v_4_2 = (cos(phi)*cos(theta)*cos(psi))*thrust/m;
v_4_3 = (cos(psi)*sin(phi)-sin(theta)*sin(psi)*cos(phi))*thrust/m;
v_4_4 = (cos(phi)*sin(theta)*cos(psi) + sin(phi)*sin(psi))/m; 

v_5_1 = (cos(psi)*(-cos(phi))-sin(theta)*sin(psi)*sin(phi))*thrust/m;
v_5_2 = (cos(theta)*sin(psi)*cos(phi))*thrust/m;
v_5_3 = (sin(theta)*cos(psi)*cos(phi)+sin(psi)*sin(phi))*thrust/m;
v_5_4 = (cos(phi)*sin(theta)*sin(psi) - sin(phi)*cos(psi))/m; 

v_6_1 = -sin(phi)*cos(theta)*thrust/m;
v_6_2 = -cos(phi)*sin(theta)*thrust/m;
v_6_3 = 0;
v_6_4 = cos(phi)*cos(theta)/m; 

V = [0 0 0 0;
     0 0 0 0;
     0 0 0 0;
    v_4_1 v_4_2 v_4_3 v_4_4;
    v_5_1 v_5_2 v_5_3 v_5_4;
    v_6_1 v_6_2 v_6_3 v_6_4];


% Uncertainties of [phi theta psi thrust] (TODO: use attitude estimator
% covariance for phi, theta, psi uncertainty)
q = [1*10^(-9) 1*10^(-9) 1*10^(-9) 3*10^(-9)];
Q = [q(1) 0 0 0;
    0 q(2) 0 0;
    0 0 q(3) 0;
    0 0 0 q(4)];


noise = [0.00003 0.00003 0.00004 0.000005]; %noise values taken from dynamic model
R = [noise(1) 0 0 0;
    0 noise(2) 0 0;
    0 0 noise(3) 0;
    0 0 0 noise(4)];


% Prediction
x_p = x + f_x * t;
sigma_p = G * sigma * G' + V*Q*V';
                                                                                %TODO
if t_act_sonar >= t_sonar
    t_act_sonar = 0;
                                                                                
    % Correction (preparation)
    if t_act_gps >= t_gps
        t_act_gps = 0;
        z_t = [ measurement(1); 
                measurement(2); 
                -measurement(3); 
                measurement(4) / sqrt(1+tan(phi)^2 + tan(theta)^2)];
    else
        z_t = [ x_p(1);
                x_p(2);
                x_p(3);
                measurement(4) / sqrt(1+tan(phi)^2 + tan(theta)^2)];
    end
    
    
    if measurement(4) >= 4.99 || measurement(4) <= 0
        z_t(4) = x_p(3);
    end
    

    h_x = [x_p(1);    %Predicted Measurement mean
           x_p(2);
           x_p(3);
           x_p(3)];

    s4_3 = sqrt(1+tan(phi)^2+tan(theta)^2);
    s4_4 = x_p(3) * 4*tan(phi)/((1+cos(2*phi)) * s4_3);
    s4_5 = x_p(3) * 4*tan(theta)/((1+cos(2*theta)) * s4_3);

    H = [ 1 0 0 0 0 0;
          0 1 0 0 0 0;
          0 0 1 0 0 0;
          0 0 1 0 0 0];

    % Correction
    K = sigma_p * H' * ( H * sigma_p * H' + R)^(-1);
    x = x_p + K * (z_t - h_x);
    sigma = (eye(6) - K * H) * sigma_p;

else
    x = x_p;
    sigma = sigma_p;
end

mu = x;
sigma_t = sigma;

== matlab function control_system/MATLAB Function ==
  data: x output; xis input; yis input; zis input; y output; z output; nodes parameter; dist output
function [x,y,z, dist] = waypoint_selector(xis, yis, zis, nodes)
%#codegen

persistent current;

if isempty(current)
    current = 1;
end

xwant = nodes(current,1);
ywant = - nodes(current,2);
zwant = - nodes(current,3);

dist = sqrt((xis-xwant)^2 + (yis-ywant)^2 + (zis-zwant)^2);
if dist < 0.6
   current = current + 1;
end

% go back
if current > size(nodes,1)
    current =  size(nodes,1)-1;
end

x = nodes(current,1);
y = - nodes(current,2);
z = - nodes(current,3);
